simulink library "INT_SmkLim_AirMsSel"  (R2016b)
settings: Solver=VariableStepAuto  StartTime=0.0  StopTime=10.0  RelTol=1e-3
settings Model: Creator=liutao  LastModifiedBy=liutao

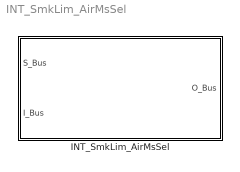
== system INT_SmkLim_AirMsSel ==
  INT_SmkLim_AirMsSel : Subsystem

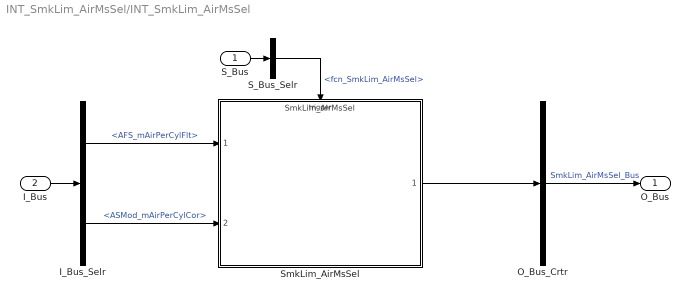
== system INT_SmkLim_AirMsSel/INT_SmkLim_AirMsSel ==
  S_Bus : Inport
  I_Bus : Inport  Port=2
  I_Bus_Selr : BusSelector  OutputSignals=AFS_mAirPerCylFlt,ASMod_mAirPerCylCor
  O_Bus_Crtr : BusCreator  Inputs=1
  S_Bus_Selr : BusSelector  OutputSignals=fcn_SmkLim_AirMsSel
  SmkLim_AirMsSel : ModelReference  ModelNameDialog=SmkLim_AirMsSel  SimulationMode=Normal  ModelReferenceVersion=1.7  TriggerPortName=function  TriggerPortTriggerType=function-call  TriggerPortStatesWhenEnabling=held
  O_Bus : Outport
  wires:
  S_Bus_Selr/1 -> SmkLim_AirMsSel/Trigger  "<fcn_SmkLim_AirMsSel>"
  S_Bus/1 -> S_Bus_Selr/1
  I_Bus/1 -> I_Bus_Selr/1
  I_Bus_Selr/1 -> SmkLim_AirMsSel/1  "<AFS_mAirPerCylFlt>"
  I_Bus_Selr/2 -> SmkLim_AirMsSel/2  "<ASMod_mAirPerCylCor>"
  O_Bus_Crtr/1 -> O_Bus/1  "SmkLim_AirMsSel_Bus"
  SmkLim_AirMsSel/1 -> O_Bus_Crtr/1
